simulink model "State feedback with kalman_Controller"  (R2021a)
settings: Solver=VariableStepAuto  StartTime=0.0  StopTime=52  RelTol=1e-3
undefined symbols (not defined in the file): A, A_d, B, B_d, C, C_d, Discrete, dt, dtref, K, kr, Lr, lr, r_i, R_kal, R_w, sigbuilder_block, Time, var
libraries: ctrlSharedLib x1
settings Model: Creator=eduma  LastModifiedBy=eduma

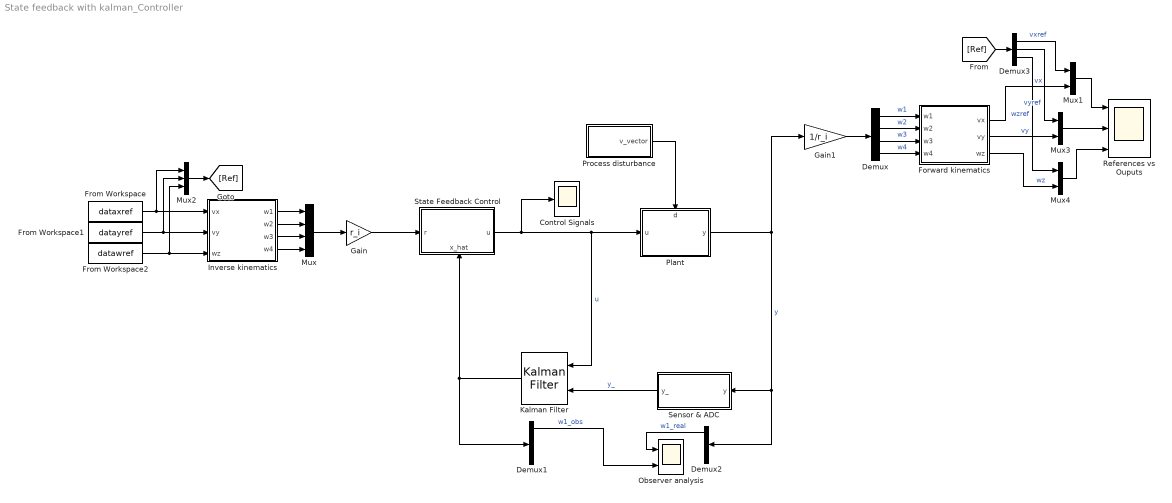
== system State feedback with kalman_Controller ==
  Control Signals : Scope
  Demux : Demux
  Demux1 : Demux  Outputs=8
  Demux2 : Demux
  Demux3 : Demux  Outputs=3
  Forward kinematics : Subsystem
  From Workspace : FromWorkspace  VariableName=dataxref  SampleTime=dtref  OutputAfterFinalValue=Setting to zero
  From Workspace1 : FromWorkspace  VariableName=datayref  SampleTime=dtref  OutputAfterFinalValue=Setting to zero
  From Workspace2 : FromWorkspace  VariableName=datawref  SampleTime=dtref  OutputAfterFinalValue=Setting to zero
  Gain : Gain  Gain=r_i
  Gain1 : Gain  Gain=1/r_i
  Inverse kinematics : Subsystem
  Kalman Filter : ctrlSharedLib/Kalman Filter  TimeDomain=Discrete-Time  UseCurrentEstimator=on  ModelSource=Individual A, B, C, D matrices  ModelSourceVariable=ss(0.95,1,1,0,1)  A=A_d  B=B_d  C=C_d  D=0  NumberOfStates=1  NumberOfInputs=1  NumberOfOutputs=1  InitialEstimateSource=Dialog  X0=0  P0=10  UseK=off  UseGH=off  NumberOfProcessNoiseInputs=1  G=1  TimeInvariantG=on  H=0  TimeInvariantH=on  Q=Q_kal  TimeInvariantQ=on  R=R_kal  TimeInvariantR=on  N=0  TimeInvariantN=on  AddInputPort=on  AddEnablePort=off  OutputEstimatedY=off  OutputP=off  Ts=-1
  Mux : Mux
  Mux1 : Mux  Inputs=2
  Mux2 : Mux  Inputs=3
  Mux3 : Mux  Inputs=2
  Mux4 : Mux  Inputs=2
  Observer analysis : Scope  NumInputPorts=2
  Plant : Subsystem
      settings: PortSchema="{\"entries\":[{\"content\":{\"sides\":[{\"content\":{\"connectorIds\":[\"In1\"]},\"type\":\"ConnectorPlacement.EquallySpacedRectSide\",\"uuid\":\"1a149f68-76ec-46f2-ab28-4834629a7be0\"},{\"content\":{\"connectorIds\":[\"Out1\"],\"side\":\"RIGHT\"},\"type\":\"ConnectorPlacement.EquallySpacedRectSide\",\"uuid\":\"5b57c582-c449-44b6-9801-7406b1fe1341\"},{\"content\":{\"connectorIds\":[\"In2\"],\"side\":\"TOP\"},\"type\":\"ConnectorPlacement.EquallySpacedRectSide\",\"uuid\":\"42451ca4-4ecd-4fe5-aba2-3c8fa4bbf5bd\"}]},\"type\":\"ConnectorPlacement.EquallySpacedConnector\",\"uuid\":\"b60914ab-a59e-4f5f-bdf2-28a80d88db04\"}],\"packageUris\":[\"http://schema.mathworks.com/mf0/Connector/R2020b\"],\"version\":\"1.0\"}"
  Process disturbance : Subsystem
  References vs Ouputs : Scope  NumInputPorts=3
  Sensor & ADC : Subsystem
  State Feedback Control : Subsystem
      settings: PortSchema="{\"entries\":[{\"content\":{\"sides\":[{\"content\":{\"connectorIds\":[\"In1\"]},\"type\":\"ConnectorPlacement.EquallySpacedRectSide\",\"uuid\":\"7310b61c-178a-46a1-82d3-74423dc4586d\"},{\"content\":{\"connectorIds\":[\"Out1\"],\"side\":\"RIGHT\"},\"type\":\"ConnectorPlacement.EquallySpacedRectSide\",\"uuid\":\"47a4d2ec-6b8c-4045-85e9-316294b7cf37\"},{\"content\":{\"connectorIds\":[],\"side\":\"TOP\"},\"type\":\"ConnectorPlacement.EquallySpacedRectSide\",\"uuid\":\"2fb50cff-bec4-4dbb-bdc8-7dff72f23688\"},{\"content\":{\"connectorIds\":[\"In2\"],\"side\":\"BOTTOM\"},\"type\":\"ConnectorPlacement.EquallySpacedRectSide\",\"uuid\":\"3763e1e5-f1b4-4eda-b68f-8c5ad54ff9b2\"}]},\"type\":\"ConnectorPlacement.EquallySpacedConnector\",\"uuid\":\"bbf162da-487a-4d6f-b474-f4b7db985ae3\"}],\"packageUris\":[\"http://schema.mathworks.com/mf0/Connector/R2020b\"],\"version\":\"1.0\"}"
  wires:
  Plant/1(y) -> Gain1/1, Demux2/1, Sensor & ADC/1(y)  "y"
  Demux/1 -> Forward kinematics/1(w1)  "w1"
  Demux/2 -> Forward kinematics/2(w2)  "w2"
  Demux/3 -> Forward kinematics/3(w3)  "w3"
  Demux/4 -> Forward kinematics/4(w4)  "w4"
  Inverse kinematics/1(w1) -> Mux/1
  Inverse kinematics/2(w2) -> Mux/2
  Inverse kinematics/3(w3) -> Mux/3
  Inverse kinematics/4(w4) -> Mux/4
  Forward kinematics/1(vx) -> Mux1/2  "vx"
  Forward kinematics/2(vy) -> Mux3/2  "vy"
  Forward kinematics/3(wz) -> Mux4/2  "wz"
  Mux/1 -> Gain/1
  Demux1/1 -> Observer analysis/2  "w1_obs"
  Demux2/1 -> Observer analysis/1  "w1_real"
  Kalman Filter/1 -> State Feedback Control/2(x_hat), Demux1/1
  Gain1/1 -> Demux/1
  Process disturbance/1(v_vector) -> Plant/2(d)
  From Workspace1/1 -> Mux2/2, Inverse kinematics/2(vy)
  From Workspace/1 -> Mux2/1, Inverse kinematics/1(vx)
  State Feedback Control/1(u) -> Plant/1(u), Kalman Filter/1, Control Signals/1  "u"
  Gain/1 -> State Feedback Control/1(r)
  From Workspace2/1 -> Inverse kinematics/3(wz), Mux2/3
  Mux2/1 -> [Ref]
  [Ref] -> Demux3/1
  Demux3/1 -> Mux1/1  "vxref"
  Mux1/1 -> References vs Ouputs/1
  Demux3/2 -> Mux3/1  "vyref"
  Demux3/3 -> Mux4/1  "wzref"
  Mux3/1 -> References vs Ouputs/2
  Mux4/1 -> References vs Ouputs/3
  Sensor & ADC/1(y_) -> Kalman Filter/2  "y_"

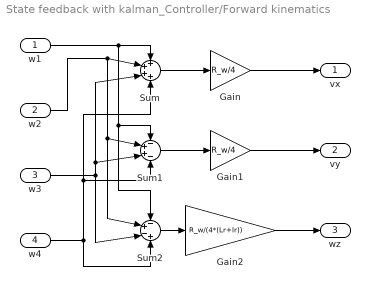
== system State feedback with kalman_Controller/Forward kinematics ==
  w1 : Inport
  w2 : Inport  Port=2
  w3 : Inport  Port=3
  w4 : Inport  Port=4
  Gain : Gain  Gain=R_w/4
  Gain1 : Gain  Gain=R_w/4
  Gain2 : Gain  Gain=R_w/(4*(Lr+lr))
  Sum : Sum  Inputs=++++
  Sum1 : Sum  Inputs=-++-
  Sum2 : Sum  Inputs=-+-+
  vx : Outport
  vy : Outport  Port=2
  wz : Outport  Port=3
  wires:
  w3/1 -> Sum/3, Sum1/3, Sum2/3
  Gain2/1 -> wz/1
  w4/1 -> Sum2/4, Sum1/4, Sum/4
  Sum2/1 -> Gain2/1
  w2/1 -> Sum2/2, Sum1/2, Sum/2
  Sum/1 -> Gain/1
  Gain1/1 -> vy/1
  w1/1 -> Sum2/1, Sum1/1, Sum/1
  Sum1/1 -> Gain1/1
  Gain/1 -> vx/1

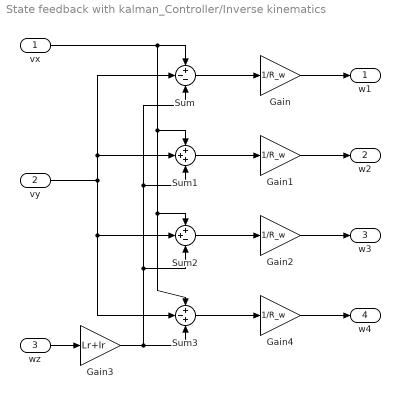
== system State feedback with kalman_Controller/Inverse kinematics ==
  vx : Inport
  vy : Inport  Port=2
  wz : Inport  Port=3
  Gain{,1..2,4} (4 alike) : Gain  Gain=1/R_w
  Gain3 : Gain  Gain=Lr+lr
  Sum : Sum  Inputs=+--
  Sum1 : Sum  Inputs=+++
  Sum2 : Sum  Inputs=++-
  Sum3 : Sum  Inputs=+-+
  w1 : Outport
  w2 : Outport  Port=2
  w3 : Outport  Port=3
  w4 : Outport  Port=4
  wires:
  Sum/1 -> Gain/1
  vx/1 -> Sum3/1, Sum2/1, Sum1/1, Sum/1
  vy/1 -> Sum1/2, Sum/2, Sum3/2, Sum2/2
  Gain3/1 -> Sum3/3, Sum/3, Sum1/3, Sum2/3
  wz/1 -> Gain3/1
  Gain/1 -> w1/1
  Gain1/1 -> w2/1
  Gain2/1 -> w3/1
  Gain4/1 -> w4/1
  Sum3/1 -> Gain4/1
  Sum2/1 -> Gain2/1
  Sum1/1 -> Gain1/1

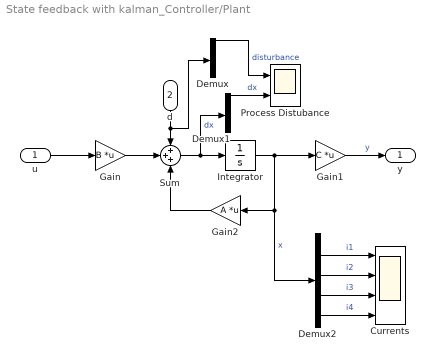
== system State feedback with kalman_Controller/Plant ==
  u : Inport
  d : Inport  Port=2
  Currents : Scope  NumInputPorts=4
  Demux : Demux  Outputs=8
  Demux1 : Demux  Outputs=8
  Demux2 : Demux  Outputs=8
  Gain : Gain  Gain=B  Multiplication=Matrix(K*u)
  Gain1 : Gain  Gain=C  Multiplication=Matrix(K*u)
  Gain2 : Gain  Gain=A  Multiplication=Matrix(K*u)
  Integrator : Integrator
  Process Distubance : Scope  NumInputPorts=2
  Sum : Sum  Inputs=+++
  y : Outport
  wires:
  u/1 -> Gain/1
  Gain/1 -> Sum/2
  Gain1/1 -> y/1  "y"
  Integrator/1 -> Demux2/1, Gain2/1, Gain1/1  "x"
  Gain2/1 -> Sum/3
  Sum/1 -> Demux1/1, Integrator/1  "dx"
  d/1 -> Demux/1, Sum/1
  Demux/1 -> Process Distubance/1  "disturbance"
  Demux1/1 -> Process Distubance/2  "dx"
  Demux2/2 -> Currents/1  "i1"
  Demux2/4 -> Currents/2  "i2"
  Demux2/6 -> Currents/3  "i3"
  Demux2/8 -> Currents/4  "i4"

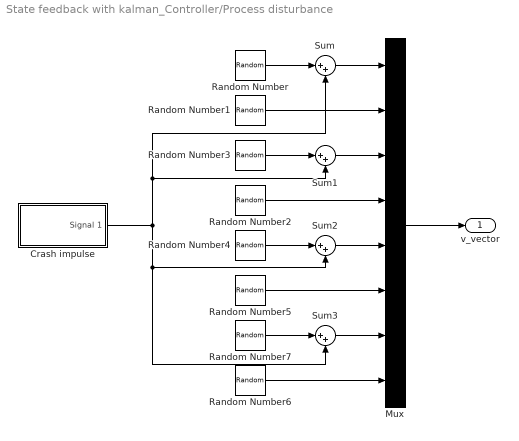
== system State feedback with kalman_Controller/Process disturbance ==
  Crash impulse : Subsystem  Tag=STV Subsys  LoadFcn=sigbuilder_block('load');  StartFcn=sigbuilder_block('start');  StopFcn=sigbuilder_block('stop');  ClipboardFcn=sigbuilder_block('clipboard');  mask(Sigbuilder block){tuvar=[0:10]}
      mask help: Simulink:masks:SigbuilderBlock_MD
      mask init:
      | if ~strcmp(get_param(bdroot(gcbh),'SimulationStatus'),'stopped') tuvar = sigbuilder_block('maskInit'); end
      settings: CopyFcn=sigbuilder_block('copy');  DeleteFcn=sigbuilder_block('delete');  ModelCloseFcn=sigbuilder_block('modelClose');  PreSaveFcn=sigbuilder_block('preSave');  PauseFcn=sigbuilder_block('pause');  ContinueFcn=sigbuilder_block('continue');  NameChangeFcn=sigbuilder_block('namechange');  OpenFcn=sigbuilder_block('open',[6 30 1248 659.25 ]);  CloseFcn=sigbuilder_block('close');
      mask Display: plot(0, 0, 100, 100,[2, 2, 32, 32, 2], [68, 8, 8, 68, 68],[32, 2], [38, 38], [32, 19, 2],[53, 60, 44], [32, 17, 17, 2],[16, 16, 31, 31]);txt = getActiveGroup(gcbh);text(2, 100, txt,'verticalAlignment', 'top');
  Mux : Mux  Inputs=8
  Random Number : RandomNumber  Variance=var  SampleTime=dt
  Random Number1 : RandomNumber  Variance=var  Seed=1  SampleTime=dt
  Random Number2 : RandomNumber  Variance=var  Seed=3  SampleTime=dt
  Random Number3 : RandomNumber  Variance=var  Seed=2  SampleTime=dt
  Random Number4 : RandomNumber  Variance=var  Seed=4  SampleTime=dt
  Random Number5 : RandomNumber  Variance=var  Seed=5  SampleTime=dt
  Random Number6 : RandomNumber  Variance=var  Seed=7  SampleTime=dt
  Random Number7 : RandomNumber  Variance=var  Seed=6  SampleTime=dt
  Sum{,1..3} (4 alike) : Sum  Inputs=|++
  v_vector : Outport
  wires:
  Random Number1/1 -> Mux/2
  Random Number3/1 -> Sum1/1
  Random Number2/1 -> Mux/4
  Random Number4/1 -> Sum2/1
  Random Number5/1 -> Mux/6
  Random Number6/1 -> Mux/8
  Mux/1 -> v_vector/1
  Random Number/1 -> Sum/1
  Sum/1 -> Mux/1
  Sum1/1 -> Mux/3
  Sum2/1 -> Mux/5
  Random Number7/1 -> Sum3/1
  Sum3/1 -> Mux/7
  Crash impulse/1(Signal 1) -> Sum2/2, Sum3/2, Sum/2, Sum1/2

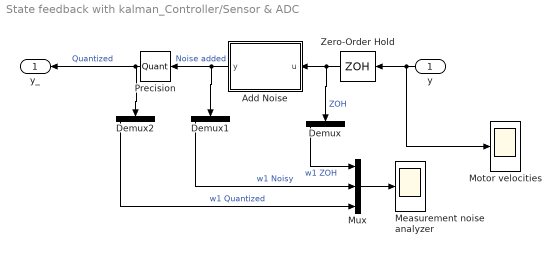
== system State feedback with kalman_Controller/Sensor & ADC ==
  y : Inport
  Add Noise : MATLAB Function  TreatAsAtomicUnit=on
  Demux : Demux
  Demux1 : Demux
  Demux2 : Demux
  Measurement noise analyzer : Scope
  Motor velocities : Scope
  Mux : Mux  Inputs=3
  Precision : Quantizer  QuantizationInterval=dw
  Zero-Order Hold : ZeroOrderHold  SampleTime=dt
  y_ : Outport
  wires:
  Add Noise/1(y) -> Demux1/1, Precision/1  "Noise added"
  Zero-Order Hold/1 -> Demux/1, Add Noise/1(u)  "ZOH"
  Precision/1 -> Demux2/1, y_/1  "Quantized"
  y/1 -> Motor velocities/1, Zero-Order Hold/1
  Mux/1 -> Measurement noise analyzer/1
  Demux/1 -> Mux/1  "w1 ZOH"
  Demux2/1 -> Mux/3  "w1 Quantized"
  Demux1/1 -> Mux/2  "w1 Noisy"

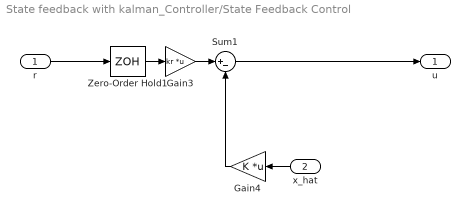
== system State feedback with kalman_Controller/State Feedback Control ==
  r : Inport
  x_hat : Inport  Port=2
  Gain3 : Gain  Gain=kr  Multiplication=Matrix(K*u)
  Gain4 : Gain  Gain=K  Multiplication=Matrix(K*u)
  Sum1 : Sum  Inputs=|+-
  Zero-Order Hold1 : ZeroOrderHold  SampleTime=dt
  u : Outport
  wires:
  x_hat/1 -> Gain4/1
  Gain3/1 -> Sum1/1
  Gain4/1 -> Sum1/2
  Zero-Order Hold1/1 -> Gain3/1
  Sum1/1 -> u/1
  r/1 -> Zero-Order Hold1/1

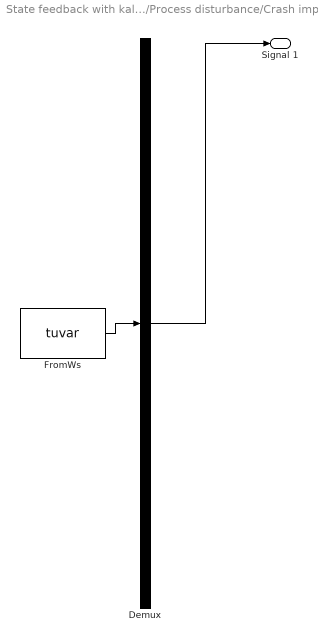
== system State feedback with kalman_Controller/Process disturbance/Crash impulse ==
  Demux : Demux  Tag=STV Demux  Outputs=1
      settings: DisplayOption=none
  FromWs : FromWorkspace  Tag=STV FromWs  VariableName=tuvar
      SigBuilderData=|
      | common.afterFinalStr = 'Extrapolate'
      | common.sampleTime = 0
      | dataSet.timeRange = [0 20]
      | dataSet.name = 'Group 1'
      | sbobj.Groups.Name = 'Group 1'
      | sbobj.Groups.Signals.Name = 'Signal 1'
      | sbobj.Groups.Signals.XData = [0 15 15 15.2 15.2 20]
      | sbobj.Groups.Signals.YData = [0 0 -40 -40 0 0]
      | sbobj.Groups.TimeRange = [0 20]
  Signal 1 : Outport  Tag=STV Outport
  wires:
  Demux/1 -> Signal 1/1
  FromWs/1 -> Demux/1

== matlab function State feedback with kalman_Controller/Sensor & ADC/Add Noise ==
  data: u input; y output
function y = fcn(u)
    y = u.*(1 + 0.05*randn(size(u)));
